simulink model "simulacao"  (R2020a)
settings: Solver=VariableStepAuto  StartTime=0.0  StopTime=10  RelTol=1e-3
values from neighbouring files (symbols this model uses):
  friction = friction.*1    [quatercar_data.m]
  g = 9.8    [quatercar_data.m]
  Jw = WHL.Inertia    [quatercar_data.m]
  M = EV.Mass    [quatercar_data.m]
  Red = 9    [quatercar_data.m]
  Rw = WHL.LoadedRadius    [quatercar_data.m]
  slip = [0 0.025 0.05 0.075 0.1 0.125 0.15 0.175 0.2 0.225 0.25 0.275 0.3 0.325 0.35 0.375 0.4 0.425 0.45 0.475 0.5 0.525 0.55 0.575 0.6 0.625 0.65 0.675 0.7 0.725 0.75 0.775 0.8 0.825 0.85 0.875 0.9 0.925 0.95 0.975 1]    [quatercar_data.m]
  Tmotor = 0.03    [quatercar_data.m]
  Tpneu = 0.001    [quatercar_data.m]
undefined symbols (not defined in the file or in its folder): EV, MTR
libraries: simulink x2
settings Model: SimulationMode=accelerator  Creator=hiked  LastModifiedBy=rodri

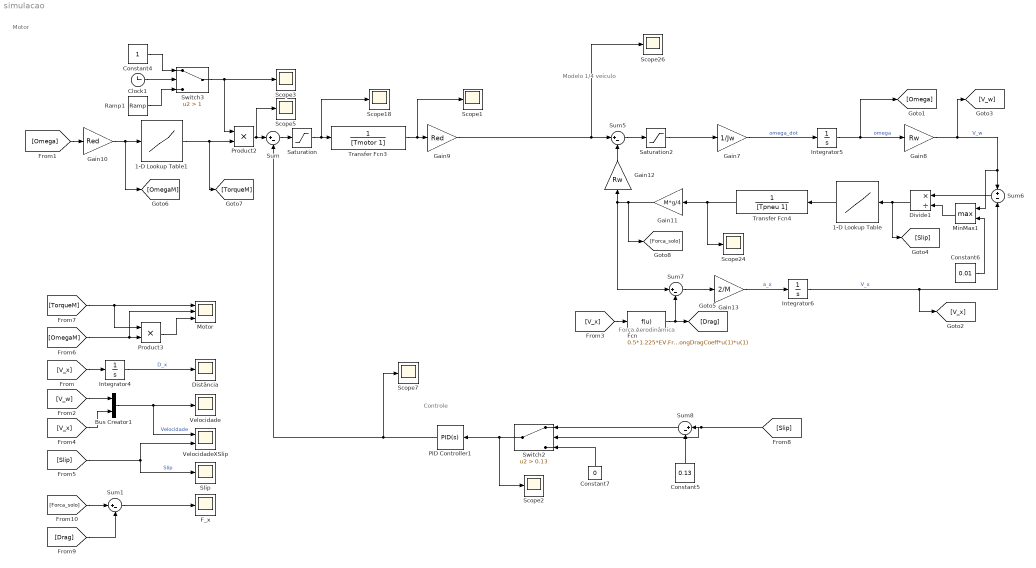
== system simulacao ==
  note: Controle
  note: Força Aerodinâmica
  note: Modelo 1/4 veículo
  note: Motor
  1-D Lookup Table : Lookup_n-D  NumberOfTableDimensions=1  BreakpointsForDimension1=slip  BreakpointsForDimension1FirstPoint=0  BreakpointsForDimension1Spacing=0.05  Table=friction  InternalRulePriority=Speed  RndMeth=Simplest  InputSameDT=on
  1-D Lookup Table1 : Lookup_n-D  NumberOfTableDimensions=1  BreakpointsForDimension1=MTR.Speed  BreakpointsForDimension1Spacing=0.25  Table=MTR.Torque*MTR.Overpower  InternalRulePriority=Speed  RndMeth=Simplest  InputSameDT=on
  Bus Creator1 : BusCreator  Inputs=2
  Clock1 : Clock
  Constant4 : Constant
  Constant5 : Constant  Value=0.13
  Constant6 : Constant  Value=0.01
  Constant7 : Constant  Value=0
  Distância : Scope
  Divide1 : Product  Inputs=*/
  F_x : Scope
  Fcn : Fcn  Expr=0.5*1.225*EV.FrontalArea*EV.LongDragCoeff*u(1)*u(1)
  Gain10 : Gain  Gain=Red
  Gain11 : Gain  Gain=M*g/4
  Gain12 : Gain  Gain=Rw
  Gain13 : Gain  Gain=2/M
  Gain7 : Gain  Gain=1/Jw
  Gain8 : Gain  Gain=Rw
  Gain9 : Gain  Gain=Red
  Integrator4 : Integrator
  Integrator5 : Integrator
  Integrator6 : Integrator
  MinMax1 : MinMax  Function=max  Inputs=2
  Motor : Scope  NumInputPorts=3
  PID Controller1 : simulink/Continuous/PID Controller  Controller=PID  Form=Parallel  TimeDomain=Continuous-time  UseExternalTs=off  SampleTime=-1  IntegratorMethod=Forward Euler  FilterMethod=Forward Euler  ControllerParametersSource=internal  P=1500  I=850  D=0  UseFilter=on  N=100  TunerSelectOption=Transfer Function Based (PID Tuner App)  InitialConditionSource=internal  InitialConditionForIntegrator=0  InitialConditionForFilter=0  DifferentiatorICPrevScaledInput=0  ExternalReset=none  TrackingMode=off  Kt=1  LimitOutput=off  UpperSaturationLimit=inf  LowerSaturationLimit=-inf  LinearizeAsGain=on  AntiWindupMode=none  Kb=1  POutMin=[]  POutMax=[]  IOutMin=[]  IOutMax=[]  DOutMin=[]  DOutMax=[]  NOutMin=[]  NOutMax=[]  SumOutMin=[]  SumOutMax=[]  SaturationOutMin=[]  SaturationOutMax=[]  PParamMin=[]  PParamMax=[]  IParamMin=[]  IParamMax=[]  DParamMin=[]  DParamMax=[]  NParamMin=[]  NParamMax=[]  KbParamMin=[]  KbParamMax=[]  KtParamMin=[]  KtParamMax=[]  KbOutMin=[]  KbOutMax=[]  KtOutMin=[]  KtOutMax=[]  IntegratorOutMin=[]  IntegratorOutMax=[]  FilterOutMin=[]  FilterOutMax=[]  SumI1OutMin=[]  SumI1OutMax=[]  SumI2OutMin=[]  SumI2OutMax=[]  SumI3OutMin=[]  SumI3OutMax=[]  SumI4OutMin=[]  SumI4OutMax=[]  SumDOutMin=[]  SumDOutMax=[]  DifferentiatorOutMin=[]  DifferentiatorOutMax=[]  FilterDiffOutCoefMin=[]  FilterDiffOutCoefMax=[]  ReciprocalOutMin=[]  ReciprocalOutMax=[]  SumDenOutMin=[]  SumDenOutMax=[]  SumNumOutMin=[]  SumNumOutMax=[]  DivideOutMin=[]  DivideOutMax=[]  UdiffTsProdOutMin=[]  UdiffTsProdOutMax=[]  NTsProdOutMin=[]  NTsProdOutMax=[]  UintegralTsProdOutMin=[]  UintegralTsProdOutMax=[]  UngainTsProdOutMin=[]  UngainTsProdOutMax=[]  IntegratorContinuousStateAttributes=''  IntegratorStateMustResolveToSignalObject=off  IntegratorRTWStateStorageClass=Auto  FilterContinuousStateAttributes=''  FilterStateMustResolveToSignalObject=off  FilterRTWStateStorageClass=Auto  ParallelPVariant=InternalParameters  IdealPVariant=Disabled  IVariant=InternalParameters  DVariant=InternalParameters  IntegratorVariant=Continuous  SatVariant=Disabled  AWVariant=Passthrough  PCopyVariant=Disabled  TRVariant=Disabled  FdbkBlocksVariant=Forward  IdealPFdbkVariant=Disabled  SatFdbkVariant=Disabled  DerivativeFilterVariant=ContFilter  NVariant=InternalParameters  NCopyVariant=Disabled  FilterICVariant=InternalICsFilter  IntegratorICVariant=InternalICs  ExternalResetVariant=Disabled  TRSumVariant=Passthrough  SumFdbkVariant=Disabled  SumVariant=Sum_PID  TsampFilterVariant=InternalTs  TsampNgainVariant=Passthrough  TsampIntegralVariant=Passthrough
  Product2 : Product
  Product3 : Product
  Ramp1 : simulink/Sources/Ramp  slope=2  start=0.5  InitialOutput=0
  Saturation : Saturate  UpperLimit=48  LowerLimit=0
  Saturation2 : Saturate  UpperLimit=1000  LowerLimit=0
  Scope{1..3,5,7,18,24,26} (8 alike) : Scope
  Slip : Scope
  Sum{,1,5,7..8} (5 alike) : Sum  Inputs=|+-
  Sum6 : Sum  Inputs=+|-
  Switch2 : Switch  Criteria=u2 > Threshold  Threshold=0.13
  Switch3 : Switch  Criteria=u2 > Threshold  Threshold=1
  Transfer Fcn3 : TransferFcn  Denominator=[Tmotor 1]
  Transfer Fcn4 : TransferFcn  Denominator=[Tpneu 1]
  Velocidade : Scope
  VelocidadeXSlip : Scope  NumInputPorts=2
  wires:
  Bus Creator1/1 -> Velocidade/1, VelocidadeXSlip/1  "Velocidade"
  Gain10/1 -> [OmegaM], 1-D Lookup Table1/1
  Transfer Fcn3/1 -> Scope1/1, Gain9/1
  Saturation2/1 -> Gain7/1
  Fcn/1 -> [Drag], Sum7/2
  Ramp1/1 -> Switch3/3
  Clock1/1 -> Switch3/2
  Integrator6/1 -> [V_x], Sum6/2  "V_x"
  Constant6/1 -> MinMax1/2
  Gain11/1 -> [Forca_solo], Sum7/1, Gain12/1
  Gain13/1 -> Integrator6/1  "a_x"
  Gain7/1 -> Integrator5/1  "omega_dot"
  Transfer Fcn4/1 -> Gain11/1, Scope24/1
  Sum5/1 -> Saturation2/1
  Integrator5/1 -> [Omega], Gain8/1  "omega"
  Constant4/1 -> Switch3/1
  Sum6/1 -> Divide1/1
  MinMax1/1 -> Divide1/2
  Gain8/1 -> [V_w], Sum6/1, MinMax1/1  "V_w"
  [Omega] -> Gain10/1
  Integrator4/1 -> Distância/1  "D_x"
  Sum7/1 -> Gain13/1
  Gain12/1 -> Sum5/2
  PID Controller1/1 -> Sum/2, Scope7/1
  Switch3/1 -> Scope3/1, Product2/1
  1-D Lookup Table1/1 -> [TorqueM], Product2/2
  Constant5/1 -> Sum8/2
  Constant7/1 -> Switch2/3
  Sum8/1 -> Switch2/1
  Switch2/1 -> Scope2/1, PID Controller1/1
  Gain9/1 -> Scope26/1, Sum5/1
  Product2/1 -> Scope5/1, Sum/1
  Saturation/1 -> Scope18/1, Transfer Fcn3/1
  [Slip] -> Switch2/2, Sum8/1
  Divide1/1 -> 1-D Lookup Table/1, [Slip]
  Sum/1 -> Saturation/1
  [V_x] -> Integrator4/1
  [V_x] -> Fcn/1
  [V_w] -> Bus Creator1/1
  [V_x] -> Bus Creator1/2
  [Slip] -> VelocidadeXSlip/2, Slip/1  "Slip"
  [OmegaM] -> Motor/2, Product3/2
  [TorqueM] -> Motor/1, Product3/1
  Product3/1 -> Motor/3
  [Forca_solo] -> Sum1/1
  [Drag] -> Sum1/2
  Sum1/1 -> F_x/1
  1-D Lookup Table/1 -> Transfer Fcn4/1
